simulink model "Even_Software_rezontor_3_layer_NN_parallel"  (R2019a)
settings: Solver=VariableStepAuto  StartTime=0.0  StopTime=inf  FixedStep=0.000001  RelTol=1e-3
settings Model: NumberOfSteps=16  Creator=vardhah  LastModifiedBy=vardhah
settings DataIOCC: ReturnWorkspaceOutputs=off
settings DebuggingCC: UnderSpecifiedDimensionMsg=warning  ArithmeticOperatorsInVariantConditions=warning

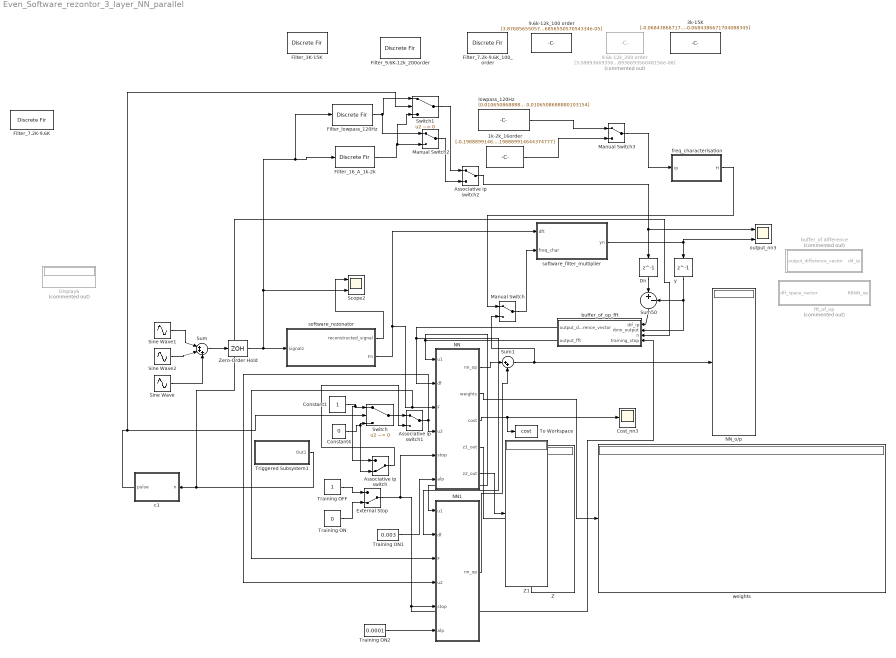
== system Even_Software_rezontor_3_layer_NN_parallel ==
  1k-2k_16order : Constant  Value=[-0.198889914644374777 0.0882189428518377339 0.0736891495871065116 0.0638368801789635787 0.0566372642221577294 0.0523172683654103132 0.0494565343907736044 0.048157521822162791 0.048157521822162791 0.0494565343907736044 0.0523172683654103132 0.0566372642221577294 0.0638368801789635787 0.0736891495871065116 0.0882189428518377339 -0.198889914644374777]  VectorParams1D=off
  3k-15K : Constant  Value=[-0.0684386671704088345 -0.0216035519389094557 -0.0869907772510868094 -0.0695372998678755599 0.0160068430386171648 -0.171506412844009415 -0.104404398490726372 0.48413102780480427 0.48413102780480427 -0.104404398490726372 -0.171506412844009415 0.0160068430386171648 -0.0695372998678755599 -0.0869907772510868094 -0.0216035519389094557 -0.0684386671704088345]  VectorParams1D=off
  9.6k-12k_100 order : Constant  Value=[3.87685655057054334e-05 0.000108803053226908729 -8.26167990877867136e-05 -0.000293336203733274498 2.6285942662608911e-05 0.000470643257144739719 0.000128704829547001234 -0.000409932472117148169 -0.000168878837800233775 5.29388077798551043e-06 -0.000285438581748162664 0.000476496961661710902 0.00138356120682394616 -0.000476433595901257331 -0.00260989841330203781 -0.000263832520003181659 0.00288776740876196033 0.00103696232298899297 -0.00148535664212565491 -0.00029781571721707251 -0.000910294888597508478 -0.00301220003423313329 0.00221471961553778218 0.00782175074594450466 -0.000709211369068674449 -0.0107696105008747954 -0.00258145844866515843 0.00855726436285330835 0.00338081517511367325 -0.00144715698429817813 0.00287506321799563301 -0.00544178445149644165 -0.016125692798747971 0.00552050119563736973 0.0291833518348223603 0.00265487109805798843 -0.0313375380418604021 -0.0109425432817974923 0.0170337904278449956 0.00463136074451602191 0.00673385154025073988 0.0271658069884841494 -0.0215094126752095813 -0.080672987166974186 0.00848125715451410883 0.135328268501058141 0.0372155688614851238 -0.164113227506699488 -0.099857601639362345 0.150463696417151488 0.150463696417151488 -0.099857601639362345 -0.164113227506699488 0.0372155688614851238 0.135328268501058141 0.00848125715451410883 -0.080672987166974186 -0.0215094126752095813 0.0271658069884841494 0.00673385154025073988 0.00463136074451602191 0.0170337904278449956 -0.0109425432817974923 -0.0313375380418604021 0.00265487109805798843 0.0291833518348223603 0.00552050119563736973 -0.016125692798747971 -0.00544178445149644165 0.00287506321799563301 -0.00144715698429817813 0.00338081517511367325 0.00855726436285330835 -0.00258145844866515843 -0.0107696105008747954 -0.000709211369068674449 0.00782175074594450466 0.00221471961553778218 -0.00301220003423313329 -0.000910294888597508478 -0.00029781571721707251 -0.00148535664212565491 0.00103696232298899297 0.00288776740876196033 -0.000263832520003181659 -0.00260989841330203781 -0.000476433595901257331 0.00138356120682394616 0.000476496961661710902 -0.000285438581748162664 5.29388077798551043e-06 -0.000168878837800233775 -0.000409932472117148169 0.000128704829547001234 0.000470643257144739719 2.6285942662608911e-05 -0.000293336203733274498 -8.26167990877867136e-05 0.000108803053226908729 3.87685655057054334e-05]  VectorParams1D=off
  9.6k-12k_200 order : Constant  Commented=on  Value=[3.58893669356048156e-08 -3.82818873463390521e-08 -2.0321720028023873e-07 4.90359188072874186e-08 5.60695246712035587e-07 1.09660540028249228e-07 -9.02554244437910404e-07 -4.11425973326973434e-07 7.02261176603049468e-07 1.84471216608655933e-07 3.26725285155721724e-07 1.85122942566739851e-06 -1.30883758906231066e-06 -6.26130099657902526e-06 3.05461039932901012e-07 1.09009807667638867e-05 3.23497432520277999e-06 -1.08958455239369133e-05 -4.97738604970975483e-06 2.96863479339988865e-06 -4.0832027868080837e-06 8.18297554751245384e-06 2.96530358064679952e-05 -9.55109847507026519e-06 -6.23922165547140565e-05 -7.71216677200245448e-06 7.59750359409520817e-05 2.93209615001356784e-05 -4.65187720652641962e-05 -1.41370609590419019e-05 -1.56985235131491563e-05 -7.53719240448361523e-05 5.59153495137252289e-05 0.000221327384655395267 -1.66050969068338295e-05 -0.000328656395451828759 -8.51260959631819787e-05 0.000282645117406031716 0.000119666235755805559 -6.72511324233616883e-05 7.71213722411986897e-05 -0.000163098688300092245 -0.000529184616157781082 0.000174782969900715956 0.000998932721197958676 0.000103789032707165716 -0.00109406787912954759 -0.000393069844497760581 0.000605548903230077127 0.00017901057135702881 0.000188671213168486616 0.0008317537932211581 -0.000616428076574026661 -0.00225801358273229787 0.000189644939633113819 0.00309786671618311488 0.000749066198738662951 -0.00246959577998202753 -0.000999305917144800888 0.000543345759446133242 -0.000591058888909330575 0.00125474640273121702 0.00385350017895572799 -0.0012819719093164299 -0.00685815514325687284 -0.000643891365732486565 0.00710257598433050412 0.00245016739238454462 -0.00372825461824609263 -0.00107354982596571057 -0.00112558364252808812 -0.00473944354418633605 0.00351472715485449472 0.0123820578712038748 -0.0011101460878915094 -0.0164148510072775998 -0.00382732465676402251 0.0127139357915301426 0.00503981617377440537 -0.00272012803122949386 0.00293385456875478335 -0.00629326791759583608 -0.0189964846306969505 0.00647240842885716226 0.0339172426787937645 0.00302977722420997957 -0.0357411919442247455 -0.0123754194694439944 0.0194465496197908511 0.00571238915438039823 0.00633940801538525594 0.0275121602229752085 -0.0219528139243238031 -0.0822938722183100269 0.00864574898877375209 0.1372509242650502 0.0376134106872798024 -0.165584050427181245 -0.100574100965544921 0.151437569678198519 0.151437569678198519 -0.100574100965544921 -0.165584050427181245 0.0376134106872798024 0.1372509242650502 0.00864574898877375209 -0.0822938722183100269 -0.0219528139243238031 0.0275121602229752085 0.00633940801538525594 0.00571238915438039823 0.0194465496197908511 -0.0123754194694439944 -0.0357411919442247455 0.00302977722420997957 0.0339172426787937645 0.00647240842885716226 -0.0189964846306969505 -0.00629326791759583608 0.00293385456875478335 -0.00272012803122949386 0.00503981617377440537 0.0127139357915301426 -0.00382732465676402251 -0.0164148510072775998 -0.0011101460878915094 0.0123820578712038748 0.00351472715485449472 -0.00473944354418633605 -0.00112558364252808812 -0.00107354982596571057 -0.00372825461824609263 0.00245016739238454462 0.00710257598433050412 -0.000643891365732486565 -0.00685815514325687284 -0.0012819719093164299 0.00385350017895572799 0.00125474640273121702 -0.000591058888909330575 0.000543345759446133242 -0.000999305917144800888 -0.00246959577998202753 0.000749066198738662951 0.00309786671618311488 0.000189644939633113819 -0.00225801358273229787 -0.000616428076574026661 0.0008317537932211581 0.000188671213168486616 0.00017901057135702881 0.000605548903230077127 -0.000393069844497760581 -0.00109406787912954759 0.000103789032707165716 0.000998932721197958676 0.000174782969900715956 -0.000529184616157781082 -0.000163098688300092245 7.71213722411986897e-05 -6.72511324233616883e-05 0.000119666235755805559 0.000282645117406031716 -8.51260959631819787e-05 -0.000328656395451828759 -1.66050969068338295e-05 0.000221327384655395267 5.59153495137252289e-05 -7.53719240448361523e-05 ...(+757 chars)]  VectorParams1D=off
  Associative ip switch : ManualSwitch  CurrentSetting=0
  Associative ip switch1 : ManualSwitch
  Associative ip switch2 : ManualSwitch
  Constant1 : Constant
  Constant4 : Constant  Value=0
  Cost_nn3 : Scope
  Display6 : Display  Commented=on
  Dn : Delay  DelayLength=1  InitialCondition=0
  External Stop : ManualSwitch  CurrentSetting=0
  Filter_16_A_1k-2k : DiscreteFir  Tag=BlockMethodSubSystem  Coefficients=[-0.198889914644374777 0.0882189428518377339 0.0736891495871065116 0.0638368801789635787 0.0566372642221577294 0.0523172683654103132 0.0494565343907736044 0.048157521822162791 0.048157521822162791 0.0494565343907736044 0.0523172683654103132 0.0566372642221577294 0.0638368801789635787 0.0736891495871065116 0.0882189428518377339 -0.198889914644374777]  InputProcessing=Columns as channels (frame based)
  Filter_3K-15K : DiscreteFir  Tag=BlockMethodSubSystem  Coefficients=[-0.0684386671704088345 -0.0216035519389094557 -0.0869907772510868094 -0.0695372998678755599 0.0160068430386171648 -0.171506412844009415 -0.104404398490726372 0.48413102780480427 0.48413102780480427 -0.104404398490726372 -0.171506412844009415 0.0160068430386171648 -0.0695372998678755599 -0.0869907772510868094 -0.0216035519389094557 -0.0684386671704088345]  InputProcessing=Columns as channels (frame based)
  "Filter_7.2K-9.6K " : DiscreteFir  Tag=BlockMethodSubSystem  Coefficients=[-0.0120785049852322399 -0.0942455273574688279 0.0101245004695954266 0.125460404555770566 0.034165372769331126 -0.1614987160724079 -0.0984930555982914957 0.150982315564688691 0.150982315564688691 -0.0984930555982914957 -0.1614987160724079 0.034165372769331126 0.125460404555770566 0.0101245004695954266 -0.0942455273574688279 -0.0120785049852322399]  InputProcessing=Columns as channels (frame based)
  Filter_7.2k-9.6K_100_order : DiscreteFir  Tag=BlockMethodSubSystem  Coefficients=[3.87685655057054334e-05 0.000108803053226908729 -8.26167990877867136e-05 -0.000293336203733274498 2.6285942662608911e-05 0.000470643257144739719 0.000128704829547001234 -0.000409932472117148169 -0.000168878837800233775 5.29388077798551043e-06 -0.000285438581748162664 0.000476496961661710902 0.00138356120682394616 -0.000476433595901257331 -0.00260989841330203781 -0.000263832520003181659 0.00288776740876196033 0.00103696232298899297 -0.00148535664212565491 -0.00029781571721707251 -0.000910294888597508478 -0.00301220003423313329 0.00221471961553778218 0.00782175074594450466 -0.000709211369068674449 -0.0107696105008747954 -0.00258145844866515843 0.00855726436285330835 0.00338081517511367325 -0.00144715698429817813 0.00287506321799563301 -0.00544178445149644165 -0.016125692798747971 0.00552050119563736973 0.0291833518348223603 0.00265487109805798843 -0.0313375380418604021 -0.0109425432817974923 0.0170337904278449956 0.00463136074451602191 0.00673385154025073988 0.0271658069884841494 -0.0215094126752095813 -0.080672987166974186 0.00848125715451410883 0.135328268501058141 0.0372155688614851238 -0.164113227506699488 -0.099857601639362345 0.150463696417151488 0.150463696417151488 -0.099857601639362345 -0.164113227506699488 0.0372155688614851238 0.135328268501058141 0.00848125715451410883 -0.080672987166974186 -0.0215094126752095813 0.0271658069884841494 0.00673385154025073988 0.00463136074451602191 0.0170337904278449956 -0.0109425432817974923 -0.0313375380418604021 0.00265487109805798843 0.0291833518348223603 0.00552050119563736973 -0.016125692798747971 -0.00544178445149644165 0.00287506321799563301 -0.00144715698429817813 0.00338081517511367325 0.00855726436285330835 -0.00258145844866515843 -0.0107696105008747954 -0.000709211369068674449 0.00782175074594450466 0.00221471961553778218 -0.00301220003423313329 -0.000910294888597508478 -0.00029781571721707251 -0.00148535664212565491 0.00103696232298899297 0.00288776740876196033 -0.000263832520003181659 -0.00260989841330203781 -0.000476433595901257331 0.00138356120682394616 0.000476496961661710902 -0.000285438581748162664 5.29388077798551043e-06 -0.000168878837800233775 -0.000409932472117148169 0.000128704829547001234 0.000470643257144739719 2.6285942662608911e-05 -0.000293336203733274498 -8.26167990877867136e-05 0.000108803053226908729 3.87685655057054334e-05]  InputProcessing=Columns as channels (frame based)
  Filter_9.6K-12k_200order : DiscreteFir  Tag=BlockMethodSubSystem  Coefficients=[3.58893669356048156e-08 -3.82818873463390521e-08 -2.0321720028023873e-07 4.90359188072874186e-08 5.60695246712035587e-07 1.09660540028249228e-07 -9.02554244437910404e-07 -4.11425973326973434e-07 7.02261176603049468e-07 1.84471216608655933e-07 3.26725285155721724e-07 1.85122942566739851e-06 -1.30883758906231066e-06 -6.26130099657902526e-06 3.05461039932901012e-07 1.09009807667638867e-05 3.23497432520277999e-06 -1.08958455239369133e-05 -4.97738604970975483e-06 2.96863479339988865e-06 -4.0832027868080837e-06 8.18297554751245384e-06 2.96530358064679952e-05 -9.55109847507026519e-06 -6.23922165547140565e-05 -7.71216677200245448e-06 7.59750359409520817e-05 2.93209615001356784e-05 -4.65187720652641962e-05 -1.41370609590419019e-05 -1.56985235131491563e-05 -7.53719240448361523e-05 5.59153495137252289e-05 0.000221327384655395267 -1.66050969068338295e-05 -0.000328656395451828759 -8.51260959631819787e-05 0.000282645117406031716 0.000119666235755805559 -6.72511324233616883e-05 7.71213722411986897e-05 -0.000163098688300092245 -0.000529184616157781082 0.000174782969900715956 0.000998932721197958676 0.000103789032707165716 -0.00109406787912954759 -0.000393069844497760581 0.000605548903230077127 0.00017901057135702881 0.000188671213168486616 0.0008317537932211581 -0.000616428076574026661 -0.00225801358273229787 0.000189644939633113819 0.00309786671618311488 0.000749066198738662951 -0.00246959577998202753 -0.000999305917144800888 0.000543345759446133242 -0.000591058888909330575 0.00125474640273121702 0.00385350017895572799 -0.0012819719093164299 -0.00685815514325687284 -0.000643891365732486565 0.00710257598433050412 0.00245016739238454462 -0.00372825461824609263 -0.00107354982596571057 -0.00112558364252808812 -0.00473944354418633605 0.00351472715485449472 0.0123820578712038748 -0.0011101460878915094 -0.0164148510072775998 -0.00382732465676402251 0.0127139357915301426 0.00503981617377440537 -0.00272012803122949386 0.00293385456875478335 -0.00629326791759583608 -0.0189964846306969505 0.00647240842885716226 0.0339172426787937645 0.00302977722420997957 -0.0357411919442247455 -0.0123754194694439944 0.0194465496197908511 0.00571238915438039823 0.00633940801538525594 0.0275121602229752085 -0.0219528139243238031 -0.0822938722183100269 0.00864574898877375209 0.1372509242650502 0.0376134106872798024 -0.165584050427181245 -0.100574100965544921 0.151437569678198519 0.151437569678198519 -0.100574100965544921 -0.165584050427181245 0.0376134106872798024 0.1372509242650502 0.00864574898877375209 -0.0822938722183100269 -0.0219528139243238031 0.0275121602229752085 0.00633940801538525594 0.00571238915438039823 0.0194465496197908511 -0.0123754194694439944 -0.0357411919442247455 0.00302977722420997957 0.0339172426787937645 0.00647240842885716226 -0.0189964846306969505 -0.00629326791759583608 0.00293385456875478335 -0.00272012803122949386 0.00503981617377440537 0.0127139357915301426 -0.00382732465676402251 -0.0164148510072775998 -0.0011101460878915094 0.0123820578712038748 0.00351472715485449472 -0.00473944354418633605 -0.00112558364252808812 -0.00107354982596571057 -0.00372825461824609263 0.00245016739238454462 0.00710257598433050412 -0.000643891365732486565 -0.00685815514325687284 -0.0012819719093164299 0.00385350017895572799 0.00125474640273121702 -0.000591058888909330575 0.000543345759446133242 -0.000999305917144800888 -0.00246959577998202753 0.000749066198738662951 0.00309786671618311488 0.000189644939633113819 -0.00225801358273229787 -0.000616428076574026661 0.0008317537932211581 0.000188671213168486616 0.00017901057135702881 0.000605548903230077127 -0.000393069844497760581 -0.00109406787912954759 0.000103789032707165716 0.000998932721197958676 0.000174782969900715956 -0.000529184616157781082 -0.000163098688300092245 7.71213722411986897e-05 -6.72511324233616883e-05 0.000119666235755805559 0.000282645117406031716 -8.51260959631819787e-05 -0.000328656395451828759 -1.66050969068338295e-05 0.000221327384655395267 5.59153495137252289e-05 -7.53719240448361523e-05 ...(+757 chars)]  InputProcessing=Columns as channels (frame based)
  Filter_lowpass_120Hz : DiscreteFir  Tag=BlockMethodSubSystem  Coefficients=[0.0106508688880103154 -0.0782130164075688084 -0.00929494835213155735 0.0642732062342344229 -0.0201897454691862474 -0.114660390364149489 0.10979296214724818 0.483668916430854023 0.483668916430854023 0.10979296214724818 -0.114660390364149489 -0.0201897454691862474 0.0642732062342344229 -0.00929494835213155735 -0.0782130164075688084 0.0106508688880103154]  InputProcessing=Columns as channels (frame based)
  Manual Switch : ManualSwitch  varsize=on
  Manual Switch2 : ManualSwitch
  Manual Switch3 : ManualSwitch
  NN : MATLAB Function  TreatAsAtomicUnit=on
  NN1 : MATLAB Function  TreatAsAtomicUnit=on
  NN_o/p : Display
  Scope2 : Scope  NumInputPorts=2
  Sine Wave : Sin  Amplitude=3  Frequency=50  SampleTime=0
  Sine Wave1 : Sin  Amplitude=3  Frequency=2000  SampleTime=0
  Sine Wave2 : Sin  Amplitude=3  Frequency=100  SampleTime=0
  Sum : Sum  Inputs=|+++
  Sum1 : Sum  Inputs=|++
  Sum50 : Sum  Inputs=|+-
  Switch : Switch  Criteria=u2 ~= 0
  Switch1 : Switch  Criteria=u2 ~= 0
  To Workspace : ToWorkspace  VariableName=cost  SampleTime=-1
      settings: Save2DSignal=2-D array (concatenate along first dimension)
  Training OFF : Constant
  Training ON : Constant  Value=0
  Training ON1 : Constant  Value=0.003
  Training ON2 : Constant  Value=0.0001
  Triggered Subsystem1 : Subsystem  TreatAsAtomicUnit=on
  Z : Display
  Z1 : Display
  Zero-Order Hold : ZeroOrderHold  SampleTime=0.0001
  buffer_of difference : MATLAB Function  Commented=on  TreatAsAtomicUnit=on
  buffer_of_op_fft : MATLAB Function  TreatAsAtomicUnit=on
  c1 : MATLAB Function  TreatAsAtomicUnit=on
  fft_of_op : MATLAB Function  Commented=on  TreatAsAtomicUnit=on
  freq_characterisation : MATLAB Function  TreatAsAtomicUnit=on
  "lowpass_120Hz " : Constant  Value=[0.0106508688880103154 -0.0782130164075688084 -0.00929494835213155735 0.0642732062342344229 -0.0201897454691862474 -0.114660390364149489 0.10979296214724818 0.483668916430854023 0.483668916430854023 0.10979296214724818 -0.114660390364149489 -0.0201897454691862474 0.0642732062342344229 -0.00929494835213155735 -0.0782130164075688084 0.0106508688880103154]  VectorParams1D=off
  output_nn3 : Scope  NumInputPorts=2
  software_filter_multiplier : MATLAB Function  TreatAsAtomicUnit=on
  software_rezonator : MATLAB Function  TreatAsAtomicUnit=on
  weights : Display
  y : Delay  DelayLength=1  InitialCondition=0
  wires:
  software_rezonator/1(reconstructed_signal) -> Scope2/1
  software_rezonator/2(Fn) -> software_filter_multiplier/1(dft), NN1/3(F), NN/3(F)
  software_filter_multiplier/1(yn) -> output_nn3/2, y/1
  Zero-Order Hold/1 -> Scope2/2, Filter_lowpass_120Hz/1, Filter_16_A_1k-2k/1, software_rezonator/1(signalz)
  Sine Wave1/1 -> Sum/1
  Sine Wave2/1 -> Sum/2
  Sine Wave/1 -> Sum/3
  Sum/1 -> Zero-Order Hold/1
  Filter_16_A_1k-2k/1 -> Switch1/3, Manual Switch2/2
  Dn/1 -> Sum50/1
  y/1 -> buffer_of_op_fft/2(rbnn_output), Sum50/2
  Manual Switch/1 -> software_filter_multiplier/2(freq_char)
  freq_characterisation/1(H) -> Manual Switch/1
  External Stop/1 -> NN1/5(stop), buffer_of_op_fft/4(training_stop), NN/5(stop)
  Training OFF/1 -> External Stop/1
  Training ON/1 -> External Stop/2
  Constant1/1 -> Switch/1, Associative ip switch/1
  Constant4/1 -> Associative ip switch/2, Switch/3
  NN/3(cost) -> To Workspace/1, Cost_nn3/1
  NN/2(weights) -> weights/1
  NN/4(z1_out) -> Z/1
  1k-2k_16order/1 -> Manual Switch3/2
  "lowpass_120Hz "/1 -> Manual Switch3/1
  Manual Switch3/1 -> freq_characterisation/1(ip)
  Triggered Subsystem1/1(Out1) -> buffer_of_op_fft/3(n), c1/1(n)
  c1/1(pulse) -> Switch/2, Switch1/2
  Switch/1 -> Associative ip switch1/1
  Associative ip switch1/1 -> NN/4(u2), NN1/4(u2)
  Associative ip switch/1 -> Associative ip switch1/2
  Associative ip switch2/1 -> output_nn3/1, Dn/1
  Switch1/1 -> Associative ip switch2/1
  Manual Switch2/1 -> Associative ip switch2/2
  NN/5(z2_out) -> Z1/1
  buffer_of_op_fft/1(output_difference_vector) -> NN/2(df), NN1/2(df)
  Sum50/1 -> buffer_of_op_fft/1(dif_ip)
  buffer_of_op_fft/2(output_fft) -> NN/1(u1), NN1/1(u1)
  Training ON1/1 -> NN/6(alp)
  Sum1/1 -> Manual Switch/2, NN_o/p/1
  NN/1(nn_op) -> Sum1/1
  NN1/1(nn_op) -> Sum1/2
  Filter_lowpass_120Hz/1 -> Manual Switch2/1, Switch1/1
  Training ON2/1 -> NN1/6(alp)

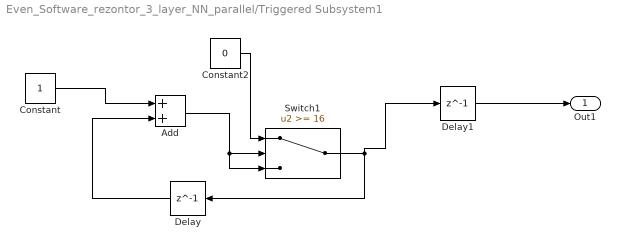
== system Even_Software_rezontor_3_layer_NN_parallel/Triggered Subsystem1 ==
  Add : Sum
  Constant : Constant
  Constant2 : Constant  Value=0
  Delay : Delay  DelayLength=1  InitialCondition=0
  Delay1 : Delay  DelayLength=1  InitialCondition=0
  Switch1 : Switch  Threshold=16
  Out1 : Outport
  wires:
  Constant2/1 -> Switch1/1
  Constant/1 -> Add/1
  Switch1/1 -> Delay1/1, Delay/1
  Delay/1 -> Add/2
  Add/1 -> Switch1/3, Switch1/2
  Delay1/1 -> Out1/1

== matlab function Even_Software_rezontor_3_layer_NN_parallel/buffer_of difference ==
  data: dif_ip input; output_difference_vector output size=[1,16]
function output_difference_vector   = difBuffer(dif_ip)                      
 
 persistent d0 d1 d2 d3 d4 d5 d6 d7 d8 d9 d10 d11 d12 d13 d14 d15;  
  
 if isempty(d0)
        d0 = 0;
 end
 if isempty(d1)
        d1 = 0;
 end
 if isempty(d2)
        d2 = 0;
 end 
 if isempty(d3)
        d3 = 0;
 end
 if isempty(d4)
        d4 = 0;
 end
 if isempty(d5)
        d5 = 0;
 end
 if isempty(d6)
        d6 = 0;
 end
 if isempty(d7)
        d7 = 0;
 end
 if isempty(d8)
        d8 = 0;
 end
 if isempty(d9)
        d9 = 0;
 end
 if isempty(d10)
        d10 = 0;
 end
 if isempty(d11)
        d11 = 0;
 end
 if isempty(d12)
        d12 = 0;
 end
 if isempty(d13)
     d13 = 0;end
 if isempty(d14)
     d14 = 0;end
 if isempty(d15)
     d15 = 0;
 end
 
 
 d15=d14;
 d14=d13;
 d13=d12;
 d12=d11;
 d11=d10;
 d10=d9;
 d9=d8;
 d8=d7;
 d7=d6;
 d6=d5;
 d5=d4;
 d4=d3; 
 d3=d2;
 d2=d1;
 d1=d0;
 d0=dif_ip;
 output_difference_vector=[d0 d1 d2 d3 d4 d5 d6 d7 d8 d9 d10 d11 d12 d13 d14 d15];

== matlab function Even_Software_rezontor_3_layer_NN_parallel/NN ==
  settings: sampleTime=0.01
  data: u1 input; df input; F input; u2 input; nn_op output; weights output; cost output; z1_out output; stop input; z2_out output; alp input
function [nn_op,weights,cost,z1_out,z2_out]  = NN(u1,df,F,u2,stop,alp)

persistent w1 w2 w3;
persistent vy;
persistent g1 g2 g3;
persistent itr;
persistent J;
persistent del_w1 del_w2 del_w3;
persistent mult1 mult2 mult3;
persistent memory_alloc_flag;
persistent r1 r2;
persistent n;

if isempty(n)
        n = 0; 
end
n=n+1;
%Important tuning parameter. 
alpha = alp;

%Hyper-parameter
M=16;   %declare batch size of training (It will also be equal to number of input in our case as we are using DFT)
E=1;    % number of external associative input

%layer declaration
input_layer =M+E; 
layer_1=16;
layer_2=256;
layer_3=16;
output_layer=layer_3;

%Allocation of multiplier ( one time execution) 
if isempty(memory_alloc_flag)
        memory_alloc_flag = 0; 
end
if isempty(mult1)
       mult1=zeros(layer_1,layer_1*input_layer); 
end
if isempty(mult2)
       mult2=zeros(layer_2,layer_1*layer_2); 
end
if isempty(mult3)
       mult3=zeros(layer_3,layer_2*layer_3); 
end
if memory_alloc_flag==0
 %write memory allocation for looped code here.It runs once and store it in memory.  
 mult1=[];
 mult2=[];
 mult3=[];
  for iteration =1:layer_1
   mult1=[mult1;[zeros(1,(iteration-1)*input_layer) ones(1,input_layer) zeros(1,(layer_1-iteration)*input_layer)]];
  end
  for iterate=1:layer_2
   mult2=[mult2;[zeros(1,(iterate-1)*layer_1) ones(1,layer_1) zeros(1,(layer_2-iterate)*layer_1)]];
  end
  for iterate=1:layer_3
   mult3=[mult3;[zeros(1,(iterate-1)*layer_2) ones(1,layer_2) zeros(1,(layer_3-iterate)*layer_2)]];
  end
 memory_alloc_flag=1;
end

%delta of weight storage
if isempty(del_w1)
    del_w1=zeros(1,input_layer*layer_1);
end
if isempty(del_w2)
    del_w2=zeros(1,layer_2*layer_1);
end
if isempty(del_w3)
    del_w3=zeros(1,layer_2*layer_3);
end

%Intialising iteration number & cost value. 
if isempty(itr)
    itr=0;
end
if isempty(J)
    J=0;
end
if isempty(r1)
    r1=0;
end
if isempty(r2)
    r2=0;
end
%gradient initialisation
if isempty(g1)
    g1= zeros(M,input_layer*layer_1);   
end
if isempty(g2)
    g2= zeros(M,layer_1*layer_2);   
end
if isempty(g3)
    g3= zeros(M,layer_3*layer_2);   
end

%prestored Vy matrix
if isempty(vy)
    vy=[0.0625000000000000,0.0625000000000000,0.0625000000000000,0.0625000000000000,0.0625000000000000,0.0625000000000000,0.0625000000000000,0.0625000000000000,0.0625000000000000,0.0625000000000000,0.0625000000000000,0.0625000000000000,0.0625000000000000,0.0625000000000000,0.0625000000000000,0.0625000000000000;0.0577424707819554,0.0441941738241592,0.0239177145228181,-1.14810637420064e-17,-0.0239177145228181,-0.0441941738241592,-0.0577424707819554,-0.0625000000000000,-0.0577424707819554,-0.0441941738241592,-0.0239177145228181,3.82702124733548e-18,0.0239177145228181,0.0441941738241592,0.0577424707819554,0.0625000000000000;0.0441941738241592,-2.67891487313484e-17,-0.0441941738241592,-0.0625000000000000,-0.0441941738241592,1.91351062366774e-17,0.0441941738241592,0.0625000000000000,0.0441941738241592,-1.14810637420064e-17,-0.0441941738241592,-0.0625000000000000,-0.0441941738241592,3.82702124733548e-18,0.0441941738241592,0.0625000000000000;0.0239177145228179,-0.0441941738241592,-0.0577424707819554,3.44431912260193e-17,0.0577424707819555,0.0441941738241592,-0.0239177145228182,-0.0625000000000000,-0.0239177145228181,0.0441941738241592,0.0577424707819554,-1.14810637420064e-17,-0.0577424707819554,-0.0441941738241592,0.0239177145228181,0.0625000000000000;-1.68427621172548e-16,-0.0625000000000000,-6.12710262471544e-17,0.0625000000000000,-1.53119536183206e-16,-0.0625000000000000,3.44431912260193e-17,0.0625000000000000,-2.67891487313484e-17,-0.0625000000000000,1.91351062366774e-17,0.0625000000000000,-1.14810637420064e-17,-0.0625000000000000,3.82702124733548e-18,0.0625000000000000;-0.0239177145228182,-0.0441941738241591,0.0577424707819554,-1.68427621172548e-16,-0.0577424707819554,0.0441941738241592,0.0239177145228181,-0.0625000000000000,0.0239177145228182,0.0441941738241592,-0.0577424707819554,1.91351062366774e-17,0.0577424707819554,-0.0441941738241592,-0.0239177145228181,0.0625000000000000;-0.0441941738241596,-3.06548562684706e-17,0.0441941738241593,-0.0625000000000000,0.0441941738241594,-1.68427621172548e-16,-0.0441941738241592,0.0625000000000000,-0.0441941738241592,3.44431912260193e-17,0.0441941738241592,-0.0625000000000000,0.0441941738241592,-1.14810637420064e-17,-0.0441941738241592,0.0625000000000000;-0.0577424707819556,0.0441941738241594,-0.0239177145228178,-3.06548562684706e-17,0.0239177145228179,-0.0441941738241591,0.0577424707819554,-0.0625000000000000,0.0577424707819555,-0.0441941738241592,0.0239177145228182,-2.67891487313484e-17,-0.0239177145228181,0.0441941738241592,-0.0577424707819554,0.0625000000000000;-0.0625000000000000,0.0625000000000000,-0.0625000000000000,0.0625000000000000,-0.0625000000000000,0.0625000000000000,-0.0625000000000000,0.0625000000000000,-0.0625000000000000,0.0625000000000000,-0.0625000000000000,0.0625000000000000,-0.0625000000000000,0.0625000000000000,-0.0625000000000000,0.0625000000000000;-0.0239177145228184,0.0441941738241592,-0.0577424707819555,0.0625000000000000,-0.0577424707819553,0.0441941738241592,-0.0239177145228180,-6.88863824520386e-17,0.0239177145228181,-0.0441941738241593,0.0577424707819554,-0.0625000000000000,0.0577424707819554,-0.0441941738241592,0.0239177145228181,0;-0.0441941738241594,0.0625000000000000,-0.0441941738241593,-3.36855242345096e-16,0.0441941738241595,-0.0625000000000000,0.0441941738241592,7.65404249467096e-17,-0.0441941738241593,0.0625000000000000,-0.0441941738241592,-3.82702124733548e-17,0.0441941738241593,-0.0625000000000000,0.0441941738241592,0;-0.0577424707819556,0.0441941738241592,0.0239177145228178,-0.0625000000000000,0.0239177145228177,0.0441941738241592,-0.0577424707819555,-3.06239072366412e-16,0.0577424707819554,-0.0441941738241592,-0.0239177145228181,0.0625000000000000,-0.0239177145228181,-0.0441941738241593,0.0577424707819554,0;-0.0625000000000000,6.13097125369412e-17,0.0625000000000000,1.37772764904077e-16,-0.0625000000000000,-3.36855242345096e-16,0.0625000000000000,9.18485099360515e-17,-0.0625000000000000,-6.88863824520386e-17,0.0625000000000000,4.59242549680257e-17,-0.0625000000000000,-2.29621274840129e-17,0.0625000000000000,0;-0.0577424707819553,-0.0441941738241594,0.0239177145228181,0.0625000000000000,0.0239177145228186,-0.0441941738241590,-0.0577424707819555,1.22542052494309e-16,0.0577424707819554,0.0441941738241593,-0.0239177145228180,-0.0625000000000000,-0.0239177145228182,0.0441941738241592,0.0577424707819554,0;-0.0441941738241587,-0.0625000000000000,-0.0441941738241588,6.13097125369412e-17,0.0441941738241588,0.0625000000000000,0.0441941738241592,1.07156594925393e-16,-0.0441941738241590,-0.0625000000000000,-0.0441941738241593,-5.35782974626967e-17,0.0441941738241592,0.0625000000000000,0.0441941738241592,0;-0.0239177145228178,-0.0441941738241593,-0.0577424707819556,-0.0625000000000000,-0.0577424707819556,-0.0441941738241594,-0.0239177145228184,-3.36855242345096e-16,0.0239177145228181,0.0441941738241592,0.0577424707819554,0.0625000000000000,0.0577424707819554,0.0441941738241593,0.0239177145228182,0;0,0,0,0,0,0,0,0,0,0,0,0,0,0,0,0];
end

%input initialisation
x_in = [real(u1(1)) real(u1(2)) real(u1(3)) real(u1(4)) real(u1(5)) real(u1(6)) real(u1(7)) real(u1(8)) real(u1(9)) imag(u1(1)) imag(u1(2)) imag(u1(3)) imag(u1(4)) imag(u1(5)) imag(u1(6)) imag(u1(7))];

%parameter intialisation 
v=transpose([x_in u2]);
if isempty(w1)
       w1=randn(input_layer,layer_1)*0.1;
end
if isempty(w2)
       w2=randn(layer_1,layer_2)*0.1;
end
if isempty(w3)
       w3=randn(layer_2,layer_3)*0.1;
end



%forward propogation
z1=w1'*v ;
a1=(1./(1+exp(-z1)));
an1=(a1-0.5);
z2=w2'*an1 ;
a2=(1./(1+exp(-z2)));
an2=(a2-0.5);
z3=w3'*an2 ;
a3=(1./(1+exp(-z3)));
an3=(a3-0.5);

z1_out=z1;
z2_out=z2;

%-------------> Backward Propogation -------->

%calculation of Nv:
da3_z3=a3.*(1-a3);
dn_a2=w3'.*repmat(da3_z3,1,layer_2);
da2_z2=a2.*(1-a2);
dn_z2= dn_a2.* repmat(transpose(da2_z2),output_layer,1);
dn_a1=dn_z2*w2';
da1_z1=a1.*(1-a1); 
dn_z1=dn_a1.*repmat(transpose(da1_z1),output_layer,1);
dn_v=dn_z1*w1';   %"This is Nv" 

%calculation of aD, A & B 
aD=transpose(F)*dn_v*vy;
A=[aD;eye(M-1) zeros(M-1,1)];
B=[transpose(F) ; zeros(M-1,M)]; 

%calculation of Nw(diff of N(v,w) wrt each weights)

dIn_3= da3_z3*transpose(a2);
dn_w3=repmat(dIn_3,1,layer_3).* mult3;

dIn_2= da2_z2*transpose(a1);
da2_w2=repmat(dIn_2,1,layer_2).* mult2;
dn_w2=dn_a2*da2_w2;

dIn_1= da1_z1*transpose(v);
da1_w1= repmat(dIn_1,1,layer_1).*mult1;
dn_w1=dn_a1*da1_w1;

%gradient updation
g3=A*g3+B*dn_w3;
g2=A*g2+B*dn_w2;
g1=A*g1+B*dn_w1;

%Training & updation at each instance
if mod(n,M)==0 && stop==0
    del_w1 =alpha*df*1*g1/M ;
    del_w2 =alpha*df*1*g2/M ;
    del_w3 =alpha*df*1*g3/M ;
    del_w_reshaped1= reshape(del_w1,[input_layer,layer_1]);
    del_w_reshaped2= reshape(del_w2,[layer_1,layer_2]);
    del_w_reshaped3= reshape(del_w3,[layer_2,layer_3]);
    w1=w1+ del_w_reshaped1;
    w2=w2+ del_w_reshaped2;
    w3=w3+ del_w_reshaped3; 
    itr=itr+1;
    J= sum(df.^2,'all')/(2*M);
end
cost=J;
weights=w1;


nn_op=an3;


end

== matlab function Even_Software_rezontor_3_layer_NN_parallel/buffer_of_op_fft ==
  data: output_difference_vector output size=[1,16]; output_fft output size=[1,16]; dif_ip input; rbnn_output input; n input; training_stop input
function [output_difference_vector,output_fft] = difBuffer(dif_ip,rbnn_output,n,training_stop)                      

 sz=16;                    % size of the dft 
 
 persistent a b;
 if isempty(a)
  a= zeros(1,sz);
 end
 if isempty(b)
  b= zeros(1,sz);
 end
 %{
 if n==159 && training_stop==0
  a=zeros(1,sz);
  b= zeros(1,sz);
else
 %}
  a= circshift(a,1);
  a(1)=dif_ip;
  b= circshift(b,1);
  b(1)=rbnn_output;
%end
 output_difference_vector=a; 
 output_fft=1/sz*fft(b); 
end

== matlab function Even_Software_rezontor_3_layer_NN_parallel/freq_characterisation ==
  data: ip input; H output
function H  = freq_character(ip)                      

dft_of_ip=fft(ip); 
size_dft=size(dft_of_ip,2)/2;
H =transpose([real(dft_of_ip(1:size_dft+1)) imag(dft_of_ip(2:size_dft))]);

end

== matlab function Even_Software_rezontor_3_layer_NN_parallel/fft_of_op ==
  data: RBNN_op input; dft_space_vector output size=[1,16]
function dft_space_vector  = difBuffer(RBNN_op)                      
 
 persistent d0 d1 d2 d3 d4 d5 d6 d7 d8 d9 d10 d11 d12 d13 d14 d15;  
  
 if isempty(d0)
        d0 = 0;
 end
 if isempty(d1)
        d1 = 0;
 end
 if isempty(d2)
        d2 = 0;
 end 
 if isempty(d3)
        d3 = 0;
 end
 if isempty(d4)
        d4 = 0;
 end
 if isempty(d5)
        d5 = 0;
 end
 if isempty(d6)
        d6 = 0;
 end
 if isempty(d7)
        d7 = 0;
 end
 if isempty(d8)
        d8 = 0;
 end
 if isempty(d9)
        d9 = 0;
 end
 if isempty(d10)
        d10 = 0;
 end
 if isempty(d11)
        d11 = 0;
 end
 if isempty(d12)
        d12 = 0;
 end
 if isempty(d13)
     d13 = 0;end
 if isempty(d14)
     d14 = 0;end
 if isempty(d15)
     d15 = 0;
 end
 
 
 d15=d14;
 d14=d13;
 d13=d12;
 d12=d11;
 d11=d10;
 d10=d9;
 d9=d8;
 d8=d7;
 d7=d6;
 d6=d5;
 d5=d4;
 d4=d3; 
 d3=d2;
 d2=d1;
 d1=d0;
 d0=RBNN_op;
 dft_space_vector=1/16*fft([d0 d1 d2 d3 d4 d5 d6 d7 d8 d9 d10 d11 d12 d13 d14 d15]);

== matlab function Even_Software_rezontor_3_layer_NN_parallel/NN1 ==
  settings: sampleTime=0.01
  data: u1 input; df input; F input; u2 input; nn_op output; stop input; alp input
function nn_op   = NN(u1,df,F,u2,stop,alp)

persistent w1 w2 w3;
persistent vy;
persistent g1 g2 g3;
persistent itr;
persistent J;
persistent del_w1 del_w2 del_w3;
persistent mult1 mult2 mult3;
persistent memory_alloc_flag;
persistent r1 r2;
persistent n;

if isempty(n)
        n = 0; 
end
n=n+1;
%Important tuning parameter. 
alpha = alp;

%Hyper-parameter
M=16;   %declare batch size of training (It will also be equal to number of input in our case as we are using DFT)
E=1;    % number of external associative input

%layer declaration
input_layer =M+E; 
layer_1=16;
layer_2=256;
layer_3=16;
output_layer=layer_3;

%Allocation of multiplier ( one time execution) 
if isempty(memory_alloc_flag)
        memory_alloc_flag = 0; 
end
if isempty(mult1)
       mult1=zeros(layer_1,layer_1*input_layer); 
end
if isempty(mult2)
       mult2=zeros(layer_2,layer_1*layer_2); 
end
if isempty(mult3)
       mult3=zeros(layer_3,layer_2*layer_3); 
end
if memory_alloc_flag==0
 %write memory allocation for looped code here.It runs once and store it in memory.  
 mult1=[];
 mult2=[];
 mult3=[];
  for iteration =1:layer_1
   mult1=[mult1;[zeros(1,(iteration-1)*input_layer) ones(1,input_layer) zeros(1,(layer_1-iteration)*input_layer)]];
  end
  for iterate=1:layer_2
   mult2=[mult2;[zeros(1,(iterate-1)*layer_1) ones(1,layer_1) zeros(1,(layer_2-iterate)*layer_1)]];
  end
  for iterate=1:layer_3
   mult3=[mult3;[zeros(1,(iterate-1)*layer_2) ones(1,layer_2) zeros(1,(layer_3-iterate)*layer_2)]];
  end
 memory_alloc_flag=1;
end

%delta of weight storage
if isempty(del_w1)
    del_w1=zeros(1,input_layer*layer_1);
end
if isempty(del_w2)
    del_w2=zeros(1,layer_2*layer_1);
end
if isempty(del_w3)
    del_w3=zeros(1,layer_2*layer_3);
end

%Intialising iteration number & cost value. 
if isempty(itr)
    itr=0;
end
if isempty(J)
    J=0;
end
if isempty(r1)
    r1=0;
end
if isempty(r2)
    r2=0;
end
%gradient initialisation
if isempty(g1)
    g1= zeros(M,input_layer*layer_1);   
end
if isempty(g2)
    g2= zeros(M,layer_1*layer_2);   
end
if isempty(g3)
    g3= zeros(M,layer_3*layer_2);   
end

%prestored Vy matrix
if isempty(vy)
    vy=[0.0625000000000000,0.0625000000000000,0.0625000000000000,0.0625000000000000,0.0625000000000000,0.0625000000000000,0.0625000000000000,0.0625000000000000,0.0625000000000000,0.0625000000000000,0.0625000000000000,0.0625000000000000,0.0625000000000000,0.0625000000000000,0.0625000000000000,0.0625000000000000;0.0577424707819554,0.0441941738241592,0.0239177145228181,-1.14810637420064e-17,-0.0239177145228181,-0.0441941738241592,-0.0577424707819554,-0.0625000000000000,-0.0577424707819554,-0.0441941738241592,-0.0239177145228181,3.82702124733548e-18,0.0239177145228181,0.0441941738241592,0.0577424707819554,0.0625000000000000;0.0441941738241592,-2.67891487313484e-17,-0.0441941738241592,-0.0625000000000000,-0.0441941738241592,1.91351062366774e-17,0.0441941738241592,0.0625000000000000,0.0441941738241592,-1.14810637420064e-17,-0.0441941738241592,-0.0625000000000000,-0.0441941738241592,3.82702124733548e-18,0.0441941738241592,0.0625000000000000;0.0239177145228179,-0.0441941738241592,-0.0577424707819554,3.44431912260193e-17,0.0577424707819555,0.0441941738241592,-0.0239177145228182,-0.0625000000000000,-0.0239177145228181,0.0441941738241592,0.0577424707819554,-1.14810637420064e-17,-0.0577424707819554,-0.0441941738241592,0.0239177145228181,0.0625000000000000;-1.68427621172548e-16,-0.0625000000000000,-6.12710262471544e-17,0.0625000000000000,-1.53119536183206e-16,-0.0625000000000000,3.44431912260193e-17,0.0625000000000000,-2.67891487313484e-17,-0.0625000000000000,1.91351062366774e-17,0.0625000000000000,-1.14810637420064e-17,-0.0625000000000000,3.82702124733548e-18,0.0625000000000000;-0.0239177145228182,-0.0441941738241591,0.0577424707819554,-1.68427621172548e-16,-0.0577424707819554,0.0441941738241592,0.0239177145228181,-0.0625000000000000,0.0239177145228182,0.0441941738241592,-0.0577424707819554,1.91351062366774e-17,0.0577424707819554,-0.0441941738241592,-0.0239177145228181,0.0625000000000000;-0.0441941738241596,-3.06548562684706e-17,0.0441941738241593,-0.0625000000000000,0.0441941738241594,-1.68427621172548e-16,-0.0441941738241592,0.0625000000000000,-0.0441941738241592,3.44431912260193e-17,0.0441941738241592,-0.0625000000000000,0.0441941738241592,-1.14810637420064e-17,-0.0441941738241592,0.0625000000000000;-0.0577424707819556,0.0441941738241594,-0.0239177145228178,-3.06548562684706e-17,0.0239177145228179,-0.0441941738241591,0.0577424707819554,-0.0625000000000000,0.0577424707819555,-0.0441941738241592,0.0239177145228182,-2.67891487313484e-17,-0.0239177145228181,0.0441941738241592,-0.0577424707819554,0.0625000000000000;-0.0625000000000000,0.0625000000000000,-0.0625000000000000,0.0625000000000000,-0.0625000000000000,0.0625000000000000,-0.0625000000000000,0.0625000000000000,-0.0625000000000000,0.0625000000000000,-0.0625000000000000,0.0625000000000000,-0.0625000000000000,0.0625000000000000,-0.0625000000000000,0.0625000000000000;-0.0239177145228184,0.0441941738241592,-0.0577424707819555,0.0625000000000000,-0.0577424707819553,0.0441941738241592,-0.0239177145228180,-6.88863824520386e-17,0.0239177145228181,-0.0441941738241593,0.0577424707819554,-0.0625000000000000,0.0577424707819554,-0.0441941738241592,0.0239177145228181,0;-0.0441941738241594,0.0625000000000000,-0.0441941738241593,-3.36855242345096e-16,0.0441941738241595,-0.0625000000000000,0.0441941738241592,7.65404249467096e-17,-0.0441941738241593,0.0625000000000000,-0.0441941738241592,-3.82702124733548e-17,0.0441941738241593,-0.0625000000000000,0.0441941738241592,0;-0.0577424707819556,0.0441941738241592,0.0239177145228178,-0.0625000000000000,0.0239177145228177,0.0441941738241592,-0.0577424707819555,-3.06239072366412e-16,0.0577424707819554,-0.0441941738241592,-0.0239177145228181,0.0625000000000000,-0.0239177145228181,-0.0441941738241593,0.0577424707819554,0;-0.0625000000000000,6.13097125369412e-17,0.0625000000000000,1.37772764904077e-16,-0.0625000000000000,-3.36855242345096e-16,0.0625000000000000,9.18485099360515e-17,-0.0625000000000000,-6.88863824520386e-17,0.0625000000000000,4.59242549680257e-17,-0.0625000000000000,-2.29621274840129e-17,0.0625000000000000,0;-0.0577424707819553,-0.0441941738241594,0.0239177145228181,0.0625000000000000,0.0239177145228186,-0.0441941738241590,-0.0577424707819555,1.22542052494309e-16,0.0577424707819554,0.0441941738241593,-0.0239177145228180,-0.0625000000000000,-0.0239177145228182,0.0441941738241592,0.0577424707819554,0;-0.0441941738241587,-0.0625000000000000,-0.0441941738241588,6.13097125369412e-17,0.0441941738241588,0.0625000000000000,0.0441941738241592,1.07156594925393e-16,-0.0441941738241590,-0.0625000000000000,-0.0441941738241593,-5.35782974626967e-17,0.0441941738241592,0.0625000000000000,0.0441941738241592,0;-0.0239177145228178,-0.0441941738241593,-0.0577424707819556,-0.0625000000000000,-0.0577424707819556,-0.0441941738241594,-0.0239177145228184,-3.36855242345096e-16,0.0239177145228181,0.0441941738241592,0.0577424707819554,0.0625000000000000,0.0577424707819554,0.0441941738241593,0.0239177145228182,0;0,0,0,0,0,0,0,0,0,0,0,0,0,0,0,0];
end

%input initialisation
x_in = [real(u1(1)) real(u1(2)) real(u1(3)) real(u1(4)) real(u1(5)) real(u1(6)) real(u1(7)) real(u1(8)) real(u1(9)) imag(u1(1)) imag(u1(2)) imag(u1(3)) imag(u1(4)) imag(u1(5)) imag(u1(6)) imag(u1(7))];

%parameter intialisation 
v=transpose([x_in u2]);
if isempty(w1)
       w1=randn(input_layer,layer_1)*0.1;
end
if isempty(w2)
       w2=randn(layer_1,layer_2)*0.1;
end
if isempty(w3)
       w3=randn(layer_2,layer_3)*0.1;
end



%forward propogation
z1=w1'*v ;
a1=(1./(1+exp(-z1)));
an1=(a1-0.5);
z2=w2'*an1 ;
a2=(1./(1+exp(-z2)));
an2=(a2-0.5);
z3=w3'*an2 ;
a3=(1./(1+exp(-z3)));
an3=(a3-0.5);

z1_out=z1;
z2_out=z2;

%-------------> Backward Propogation -------->

%calculation of Nv:
da3_z3=a3.*(1-a3);
dn_a2=w3'.*repmat(da3_z3,1,layer_2);
da2_z2=a2.*(1-a2);
dn_z2= dn_a2.* repmat(transpose(da2_z2),output_layer,1);
dn_a1=dn_z2*w2';
da1_z1=a1.*(1-a1); 
dn_z1=dn_a1.*repmat(transpose(da1_z1),output_layer,1);
dn_v=dn_z1*w1';   %"This is Nv" 

%calculation of aD, A & B 
aD=transpose(F)*dn_v*vy;
A=[aD;eye(M-1) zeros(M-1,1)];
B=[transpose(F) ; zeros(M-1,M)]; 

%calculation of Nw(diff of N(v,w) wrt each weights)

dIn_3= da3_z3*transpose(a2);
dn_w3=repmat(dIn_3,1,layer_3).* mult3;

dIn_2= da2_z2*transpose(a1);
da2_w2=repmat(dIn_2,1,layer_2).* mult2;
dn_w2=dn_a2*da2_w2;

dIn_1= da1_z1*transpose(v);
da1_w1= repmat(dIn_1,1,layer_1).*mult1;
dn_w1=dn_a1*da1_w1;

%gradient updation
g3=A*g3+B*dn_w3;
g2=A*g2+B*dn_w2;
g1=A*g1+B*dn_w1;

%Training & updation at each instance
if mod(n,M)==0 && stop==0
    del_w1 =alpha*df*1*g1/M ;
    del_w2 =alpha*df*1*g2/M ;
    del_w3 =alpha*df*1*g3/M ;
    del_w_reshaped1= reshape(del_w1,[input_layer,layer_1]);
    del_w_reshaped2= reshape(del_w2,[layer_1,layer_2]);
    del_w_reshaped3= reshape(del_w3,[layer_2,layer_3]);
    w1=w1+ del_w_reshaped1;
    w2=w2+ del_w_reshaped2;
    w3=w3+ del_w_reshaped3; 
    itr=itr+1;
    J= sum(df.^2,'all')/(2*M);
end
cost=J;
weights=w1;


nn_op=an3;


end

== matlab function Even_Software_rezontor_3_layer_NN_parallel/software_rezonator ==
  data: signalz input; reconstructed_signal output; Fn output size=16
function [reconstructed_signal,Fn]   = rezonator(signalz)

persistent numberofrezonator;
persistent g c bfr_rezo_sm aft_delay dft_out;
persistent out signal_dif;
persistent n;
persistent memory_alloc_flag;


%assign the number of rezonator here. For configuring it for higher order
%rezonator  we need to change (1) 'numberofrezonaotor' variable
if isempty(numberofrezonator)
        numberofrezonator = 16;   %here 16 parallel rezonators
end

%Initialisation of memory allocations/variables ====> 
if isempty(memory_alloc_flag)
        memory_alloc_flag = 0; 
end
if isempty(g)
       g=zeros(numberofrezonator,numberofrezonator,'like',0i); 
end
if isempty(c)
       c=zeros(numberofrezonator,numberofrezonator,'like',0i); 
end
if memory_alloc_flag==0
 for i=0:numberofrezonator-1
  for j= 0:numberofrezonator-1
   g(i+1,j+1)=1/numberofrezonator*(exp(-1i*2*pi*i*j/numberofrezonator));
   c(i+1,j+1)=(exp(1i*2*pi*i*j/numberofrezonator));
  end 
 end
 memory_alloc_flag=1;
end


%Initialisation of variables  =====> 
if isempty(n)
        n = 0;   
end 
if isempty(out)
  out=0+0i;
end
if isempty(signal_dif)
  signal_dif=0+0i;
end
if isempty(bfr_rezo_sm)
  bfr_rezo_sm=repmat(0+0i,numberofrezonator,1);
end
if isempty(aft_delay)
  aft_delay=repmat(0+0i,numberofrezonator,1);
end
if isempty(dft_out)
  dft_out=repmat(0+0i,numberofrezonator,1);
end

%creating cycle of rotation for selection of correct column of g & c.
cycle=mod(n,numberofrezonator);

%resonator core -----------------------------> 
dft_out=c(:,cycle+1).*aft_delay;
out= sum(dft_out,1);
signal_dif=signalz-out;
bfr_rezo_sm=g(:,cycle+1).*signal_dif;

%counting the counter
n=n+1;

% output assignment ------------------>
reconstructed_signal=out;
dft=aft_delay; 
N=size(dft,1);
a=1:1:N/2-1;
b=N/2+1:1:N-1;
dft_trans=transpose(dft);
Fn=transpose([real(dft_trans(1)) 2*(real(dft_trans(2:N/2)).*cos(2*pi*a*n/N)-imag(dft_trans(2:N/2)).*sin(2*pi*a*n/N)) -1^n*real(dft_trans(N/2+1)) -2*(imag(dft_trans(N/2+2:N)).*cos(2*pi*b*n/N)+real(dft_trans(N/2+2:N)).*sin(2*pi*b*n/N))]);
%--------output assignment over----------<

%final updation of buffer ------>>>>>>>>>>>>
aft_delay= aft_delay+bfr_rezo_sm; 
end

== matlab function Even_Software_rezontor_3_layer_NN_parallel/software_filter_multiplier ==
  data: dft input; yn output; freq_char input
function yn = fcn(dft,freq_char)
yn=transpose(freq_char)*dft;
end

== matlab function Even_Software_rezontor_3_layer_NN_parallel/c1 ==
  data: n input; pulse output
function pulse   = fcn(n)
persistent cnt;
if isempty(cnt)
    cnt=0;
end

if n==15
     cnt=cnt+1;
 end
 pulse = mod(cnt,2);
end
